simulink model "test"  (R2020b)
settings: Solver=VariableStepAuto  StartTime=0.0  StopTime=10.0  RelTol=1e-3
libraries: simulink x2
settings Model: Creator=ZIN  LastModifiedBy=ZIN

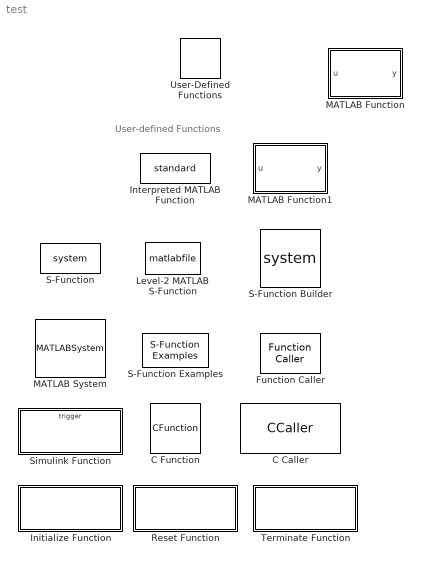
== system test ==
  note: User-defined Functions
  C Caller : CCaller
  C Function : CFunction
  Function Caller : FunctionCaller  FunctionPrototype=y = f(u)  InputArgumentSpecifications=<Enter example>  OutputArgumentSpecifications=<Enter example>
  Initialize Function : Subsystem  TreatAsAtomicUnit=on
  Interpreted MATLAB Function : MATLABFcn  MATLABFcn=standard
  Level-2 MATLAB S-Function : M-S-Function
  MATLAB Function : MATLAB Function  TreatAsAtomicUnit=on
  MATLAB Function1 : MATLAB Function  TreatAsAtomicUnit=on
  MATLAB System : MATLABSystem
  Reset Function : Subsystem  TreatAsAtomicUnit=on
  S-Function : S-Function  SFunctionDeploymentMode=off  EnableBusSupport=off
  S-Function Builder : S-Function  SFunctionDeploymentMode=off  EnableBusSupport=off  mask(S-Function Builder){}
      mask help: Simulink:masks:SFunctionBuilder_MD
      mask init:
      | val = [[.9  0.75 0.75 1 1 .9 .9 1]',[1 1 0.75 0.75 .9 .9 1 .9]'];try , sys = get_param(gcb,'SfunBuilderFcnName');if isempty(sys), sys = get_param(gcb,'FunctionName'); end,catch, sys = get_param(gcb,'FunctionName'); end
      settings: CopyFcn=set_param(gcbh,'LinkStatus','none')  OpenFcn=sfunctionwizard(gcbh)
      mask Display: plot(val(:,1),val(:,2)),disp(sys),port_label('input',1,'u0'),port_label('output',1,'y0')
  S-Function Examples : simulink/User-Defined Functions/S-Function Examples
      settings: SourceProductBaseCode=SL
  Simulink Function : Subsystem  TreatAsAtomicUnit=on
  Terminate Function : Subsystem  TreatAsAtomicUnit=on
  User-Defined Functions : simulink/User-Defined Functions  SystemSampleTime=-1  VariantActivationTime=update diagram  Latency=0  AutoFrameSizeCalculation=off
      settings: SourceProductBaseCode=SL
  wires:
  ? -> MATLAB Function/1(u)

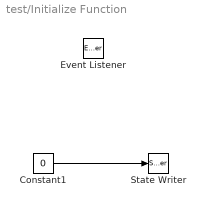
== system test/Initialize Function ==
  Constant1 : Constant  Value=0
  Event Listener : EventListener  DisableCoverage=on  EventName=reset
  State Writer : StateWriter
  wires:
  Constant1/1 -> State Writer/1

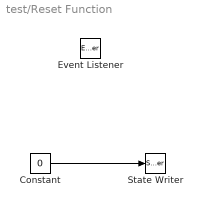
== system test/Reset Function ==
  Constant : Constant  Value=0
  Event Listener : EventListener  DisableCoverage=on  EventType=Reset  EventName=reset
  State Writer : StateWriter
  wires:
  Constant/1 -> State Writer/1

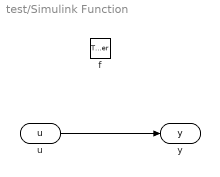
== system test/Simulink Function ==
  f : TriggerPort  TriggerType=function-call  IsSimulinkFunction=on  FunctionName=f  FunctionVisibility=scoped  VariantControl=(inherit)
  u : ArgIn  DisableCoverage=on  ArgumentName=u
  y : ArgOut  DisableCoverage=on  ArgumentName=y
  wires:
  u/1 -> y/1

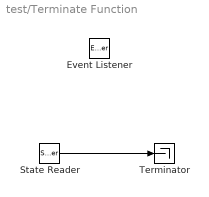
== system test/Terminate Function ==
  Event Listener : EventListener  DisableCoverage=on  EventType=Terminate  EventName=reset
  State Reader : StateReader
  Terminator : Terminator
  wires:
  State Reader/1 -> Terminator/1

== matlab function test/MATLAB Function1 ==
  data: u input; y output
function y = fcn(u)
    y = u;
end
function y = fdcn(u)
    y = u;
end

== matlab function test/MATLAB Function ==
  data: u input; y output
function y = fcn(u)

y = u;
